simulink model "sim7"  (R2022b)
settings: Solver=VariableStepAuto  StartTime=0.0  StopTime=800  RelTol=1e-10
values from neighbouring files (symbols this model uses):
  Kc = 1*tau*(0.9+td/(12*tau))/(K*td)    [lab7_221147.m]
  Ti = td*(30+3*td/tau)/(9+20*td/tau)    [lab7_221147.m]
settings Model: Creator=Administrator  LastModifiedBy=Administrator

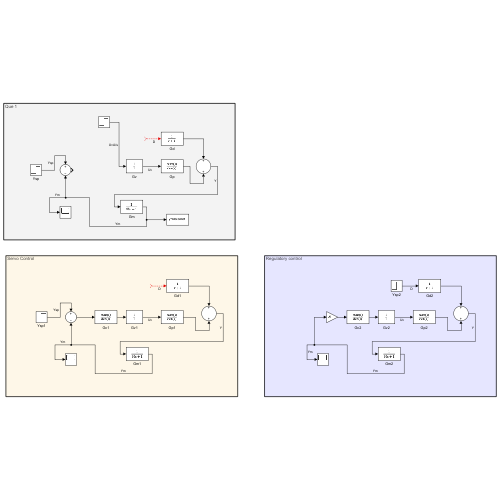
[thumbnail: Simulink's stored preview of the top-level diagram]
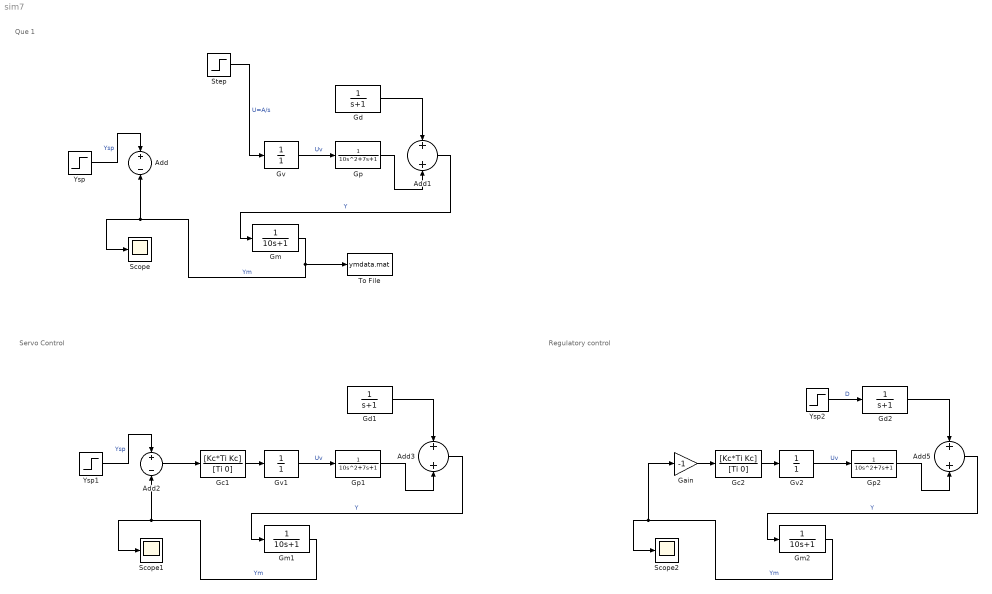
== system sim7 ==
  note: Que 1
  note: Servo Control
  note: Regulatory control
  Add : Sum  Inputs=+-
  Add1 : Sum
  Add2 : Sum  Inputs=+-
  Add3 : Sum
  Add5 : Sum
  Gain : Gain  Gain=-1
  Gc1 : TransferFcn  Numerator=[Kc*Ti Kc]  Denominator=[Ti 0]
  Gc2 : TransferFcn  Numerator=[Kc*Ti Kc]  Denominator=[Ti 0]
  Gd : TransferFcn  Denominator=[1 1]
  Gd1 : TransferFcn  Denominator=[1 1]
  Gd2 : TransferFcn  Denominator=[1 1]
  Gm : TransferFcn  Denominator=[10 1]
  Gm1 : TransferFcn  Denominator=[10 1]
  Gm2 : TransferFcn  Denominator=[10 1]
  Gp : TransferFcn  Denominator=[10 7 1]
  Gp1 : TransferFcn  Denominator=[10 7 1]
  Gp2 : TransferFcn  Denominator=[10 7 1]
  Gv : TransferFcn  Denominator=[1]
  Gv1 : TransferFcn  Denominator=[1]
  Gv2 : TransferFcn  Denominator=[1]
  Scope : Scope
  Scope1 : Scope
  Scope2 : Scope
  Step : Step  SampleTime=0
  To File : ToFile  Filename=ymdata.mat
  Ysp : Step  SampleTime=0
  Ysp1 : Step  SampleTime=0
  Ysp2 : Step  SampleTime=0
  wires:
  Add1/1 -> Gm/1  "Y"
  Gd/1 -> Add1/1
  Gv/1 -> Gp/1  "Uv"
  Gp/1 -> Add1/2
  Step/1 -> Gv/1  "U=A/s"
  Ysp/1 -> Add/1  "Ysp"
  Gm/1 -> To File/1, Scope/1, Add/2  "Ym"
  ? -> Gd/1  "D"
  ? -> Gd1/1  "D"
  Ysp1/1 -> Add2/1  "Ysp"
  Gp1/1 -> Add3/2
  Gd1/1 -> Add3/1
  Add3/1 -> Gm1/1  "Y"
  Gm1/1 -> Scope1/1, Add2/2  "Ym"
  Gv1/1 -> Gp1/1  "Uv"
  Add2/1 -> Gc1/1
  Gc1/1 -> Gv1/1
  Gm2/1 -> Gain/1, Scope2/1  "Ym"
  Gain/1 -> Gc2/1
  Gv2/1 -> Gp2/1  "Uv"
  Gp2/1 -> Add5/2
  Ysp2/1 -> Gd2/1  "D"
  Add5/1 -> Gm2/1  "Y"
  Gd2/1 -> Add5/1
  Gc2/1 -> Gv2/1
